simulink model "SIMULINK_Module"  (R2025a)
settings: Solver=VariableStepAuto  StartTime=0.0  StopTime=120  RelTol=1e-3
values from neighbouring files (symbols this model uses):
  A = zeros(10,10)    [LQR_SIMULINK.m]
  B = zeros(10,3)    [LQR_SIMULINK.m]
  C = eye(10,10)    [LQR_SIMULINK.m]
  D = zeros(10,3)    [LQR_SIMULINK.m]
  gimbal_Max = deg2rad(15)    [LQR_SIMULINK.m]
  gimbal_Min = deg2rad(-15)    [LQR_SIMULINK.m]
  max_Thrust = 11.77    [LQR_SIMULINK.m]
  min_Thrust = 0    [LQR_SIMULINK.m]
  S = zeros(10,1)    [LQR_SIMULINK.m]
  x0 = zeros(10,1)    [LQR_SIMULINK.m]
undefined symbols (not defined in the file or in its folder): K
settings Model: Creator=Hackn  LastModifiedBy=Hackn

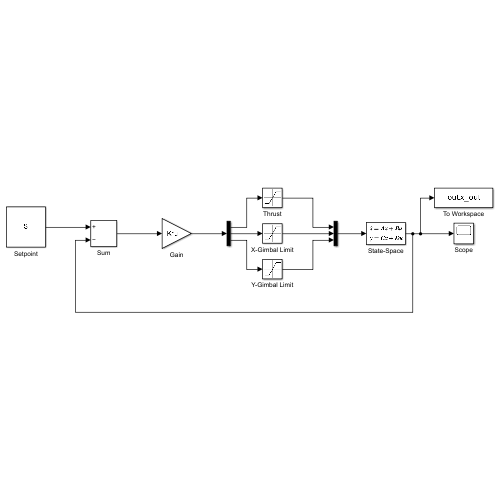
[thumbnail: Simulink's stored preview of the top-level diagram]
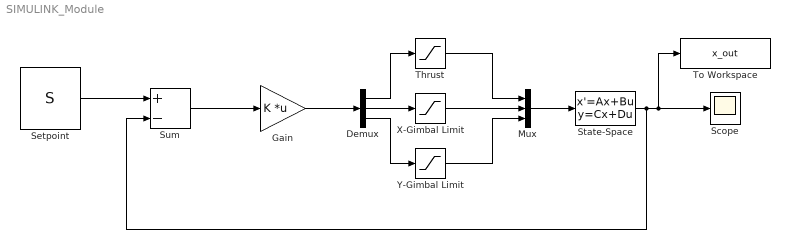
== system SIMULINK_Module ==
  Demux : Demux  Outputs=3
  Gain : Gain  Gain=K  Multiplication=Matrix(K*u)
  Mux : Mux  Inputs=3
  Scope : Scope
      settings: ActiveDisplayYMinimum=-3.34965538999647E+6  ActiveDisplayYMaximum=1.9506784440344002E+6
  Setpoint : Constant  Value=S
  State-Space : StateSpace  A=A  B=B  C=C  D=D  InitialCondition=x0
  Sum : Sum  Inputs=+-
  Thrust : Saturate  UpperLimit=max_Thrust  LowerLimit=min_Thrust
  To Workspace : ToWorkspace  VariableName=x_out  SaveFormat=Structure With Time  SampleTime=-1
  X-Gimbal Limit : Saturate  UpperLimit=gimbal_Max  LowerLimit=gimbal_Min
  Y-Gimbal Limit : Saturate  UpperLimit=gimbal_Max  LowerLimit=gimbal_Min
  wires:
  Setpoint/1 -> Sum/1
  Sum/1 -> Gain/1
  Gain/1 -> Demux/1
  Demux/1 -> Thrust/1
  Demux/2 -> X-Gimbal Limit/1
  Demux/3 -> Y-Gimbal Limit/1
  X-Gimbal Limit/1 -> Mux/2
  Thrust/1 -> Mux/1
  Y-Gimbal Limit/1 -> Mux/3
  Mux/1 -> State-Space/1
  State-Space/1 -> Sum/2, Scope/1, To Workspace/1
